simulink model "S1File_JL2005S"  (R2017a)
settings: Solver=ode8  StartTime=0.0  StopTime=96  FixedStep=1  RelTol=1e-3
libraries: cstblocks x1
settings Model: Creator=ac8227  LastModifiedBy=ac8227

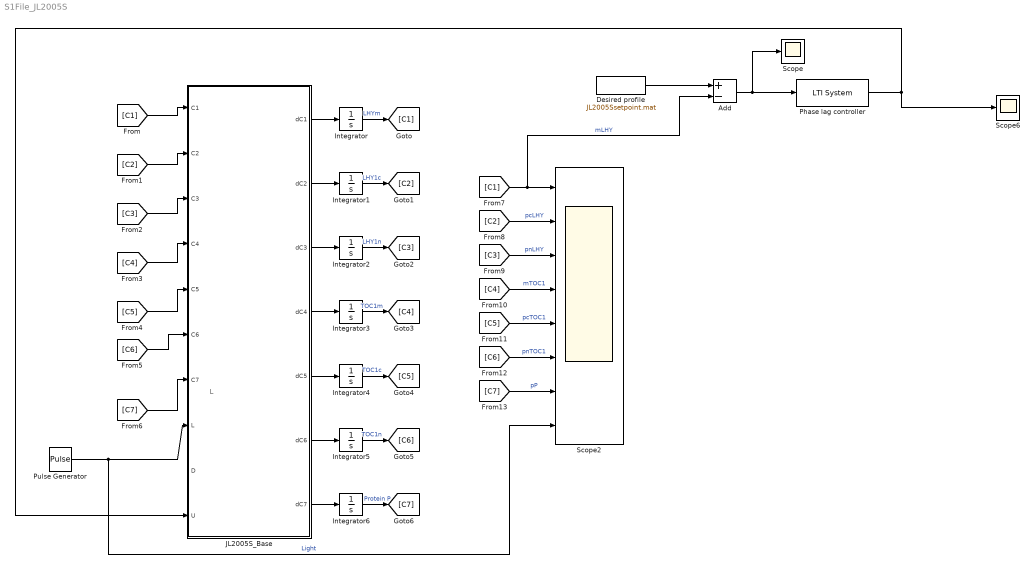
== system S1File_JL2005S ==
  note: L
  Add : Sum  Inputs=+-
  Desired profile : FromFile  FileName=JL2005Ssetpoint.mat  SampleTime=0
  Integrator : Integrator  InitialCondition=2.4051
  Integrator1 : Integrator  InitialCondition=1.3471
  Integrator2 : Integrator  InitialCondition=0.7448
  Integrator3 : Integrator  InitialCondition=0.0591
  Integrator4 : Integrator  InitialCondition=0.7377
  Integrator5 : Integrator  InitialCondition=1.3882
  Integrator6 : Integrator  InitialCondition=0.1462
  JL2005S_Base : MATLAB Function  TreatAsAtomicUnit=on
  Phase lag controller : cstblocks/LTI System  sys=tf(0.9,[1 0.026])  IC=[]
  Pulse Generator : DiscretePulseGenerator  PulseType=Time based  Period=24  PulseWidth=50
  Scope : Scope
  Scope2 : Scope  NumInputPorts=8
  Scope6 : Scope
  wires:
  JL2005S_Base/1(dC1) -> Integrator/1
  JL2005S_Base/2(dC2) -> Integrator1/1
  JL2005S_Base/3(dC3) -> Integrator2/1
  JL2005S_Base/4(dC4) -> Integrator3/1
  JL2005S_Base/5(dC5) -> Integrator4/1
  JL2005S_Base/6(dC6) -> Integrator5/1
  JL2005S_Base/7(dC7) -> Integrator6/1
  Integrator/1 -> [C1]  "LHYm"
  [C2] -> JL2005S_Base/2(C2)
  Integrator2/1 -> [C3]  "LHY1n"
  Integrator3/1 -> [C4]  "TOC1m"
  Integrator5/1 -> [C6]  "TOC1n"
  [C3] -> JL2005S_Base/3(C3)
  [C4] -> JL2005S_Base/4(C4)
  [C5] -> JL2005S_Base/5(C5)
  [C7] -> JL2005S_Base/7(C7)
  Pulse Generator/1 -> JL2005S_Base/8(L), Scope2/8  "Light"
  Integrator1/1 -> [C2]  "LHY1c"
  Integrator4/1 -> [C5]  "TOC1c"
  Integrator6/1 -> [C7]  "Protein P"
  [C2] -> Scope2/2  "pcLHY"
  [C3] -> Scope2/3  "pnLHY"
  [C4] -> Scope2/4  "mTOC1"
  [C5] -> Scope2/5  "pcTOC1"
  [C6] -> Scope2/6  "pnTOC1"
  [C7] -> Scope2/7  "pP"
  [C1] -> JL2005S_Base/1(C1)
  [C1] -> Add/2, Scope2/1  "mLHY"
  Desired profile/1 -> Add/1
  Add/1 -> Scope/1, Phase lag controller/1
  [C6] -> JL2005S_Base/6(C6)
  Phase lag controller/1 -> JL2005S_Base/10(U), Scope6/1

== matlab function S1File_JL2005S/JL2005S_Base ==
  data: C1 input; dC1 output; C2 input; C3 input; C4 input; C5 input; C6 input; C7 input; L input; dC2 output; dC3 output; dC4 output; dC5 output; dC6 output; dC7 output; D input; U input
function [dC1,dC2,dC3,dC4,dC5,dC6,dC7] = fcn(C1,C2,C3,C4,C5,C6,C7,L,D,U)

% % Base level (MSE = 0.0117)
prmLHY = [4.6322,1.4203,1.3448,1.2854];
prpcLHY = [0.4079,2.0739,1.7424];
prpnLHY = [0.93366,1.7405,1.4008];
prmTOC1 = [0.050646,-1.4632,1.4907];
prpcTOC1 = [2.4345,1.9354,0.20909];
prpnTOC1 = [0.037946,1.146,0.027235];
prpP = [0.41457,0.49865,1.6192];  

% % Range of ~50 (MSE = 0.0137)
% prmLHY = [5.4894,1.5496,1.5756,1.5542]; % Converges
% prpcLHY = [0.43143,1.9749,1.7121];
% prpnLHY = [0.95281,1.6789,1.3811];
% prmTOC1 = [0.0549,-1.4271,1.4981];
% prpcTOC1 = [2.4462,2.0075,0.194];
% prpnTOC1 = [0.037926,1.1027,0.027513];
% prpP = [0.43959,0.51775,1.656];

% % Range of ~5 (MSE = 0.0145)
% prmLHY = [5.2527,1.5661,1.7843,1.6454]; % Converges
% prpcLHY = [0.42233,2.0043,1.7272];
% prpnLHY = [0.9504,1.7281,1.3928];
% prmTOC1 = [0.058326,-1.3621,1.4769];
% prpcTOC1 = [2.3108,1.988,0.1901];
% prpnTOC1 = [0.038066,1.0268,0.027074];
% prpP = [0.43225,0.50767,1.6472];

% % Range of ~0.5 (MSE = 0.0110)
% prmLHY = [3.0747,1.3927,1.1786,1.2202]; % Converges
% prpcLHY = [0.3659,2.6423,2.0228];
% prpnLHY = [0.93817,1.8163,1.4234];
% prmTOC1 = [0.055651,-1.2895,1.3695];
% prpcTOC1 = [2.4229,1.9556,0.21217];
% prpnTOC1 = [0.037499,1.0855,0.026666];
% prpP = [0.41153,0.4926,1.4557];

% % Range of ~0.05 (MSE = 0.0692) % Doesn't reproduce the data
% prmLHY = [4.6016,1.3393,0.050877,0.92426];
% prpcLHY = [0.42702,2.1766,1.7808];
% prpnLHY = [0.959,1.8974,1.3132];
% prmTOC1 = [0.049209,-1.5428,1.4638];
% prpcTOC1 = [2.591,1.9552,0.21885];
% prpnTOC1 = [0.039229,1.1923,0.028089];
% prpP = [0.4147,0.51645,1.5603];

theta = [prmLHY prpcLHY prpnLHY prmTOC1 prpcTOC1 prpnTOC1 prpP];


% % mLHY
% dC1 = real(theta(1)*C6^(theta(2)) - theta(3)*C1 + theta(4)*C7*L);
% 
% % pcLHY
% dC2 = real(theta(5)*C1^(theta(6)) - theta(7)*C2);
% 
% % pnLHY
% dC3 = real(theta(8)*C2^(theta(9)) - theta(10)*C3);
% 
% % mTOC1
% dC4 = real(theta(11)*C3^(theta(12)) - theta(13)*C4);
% 
% % pcTOC1
% dC5 = real(theta(14)*C4^(theta(15)) - theta(16)*C5);
% 
% % pnTOC1
% dC6 = real(theta(17)*C5^(theta(18)) - theta(19)*C6 + D);
% 
% % pP
% dC7 = real(theta(20)*(1-L) - theta(21)*C7 + theta(22)*C7*L);

% LHY mRNA
% dC1 = theta(1)*C7*L + theta(2)*C6^(theta(3)*0)*U - theta(4)*C1;
dC1 = theta(1)*C7*L + theta(2)*U^(theta(3)) - theta(4)*C1;

% LHY protein cytosol
dC2 = theta(5)*C1^theta(6) - theta(7)*C2;

% LHY protein nucleus
dC3 = theta(8)*C2^theta(9) - theta(10)*C3;

% TOC1 mRNA
dC4 = theta(11)*C3^theta(12) - theta(13)*C4;

% TOC1 protein cytosol
dC5 = theta(14)*C4^theta(15) - theta(16)*C5;

% TOC1 protein nucleus
dC6 = theta(17)*C5^theta(18) - theta(19)*C6 + 0*D;

% Protein P
dC7 = theta(20)*(1 - L) - theta(21)*C7 - theta(22)*L*C7;
